simulink model "model"  (R2022b)
settings: Solver=VariableStepAuto  StartTime=0.0  StopTime=10.0  RelTol=1e-3
values from neighbouring files (symbols this model uses):
  a32 = A(3,2)    [parametry.m]
  a33 = A(3,3)    [parametry.m]
  a34 = A(3,4)    [parametry.m]
  a42 = A(4,2)    [parametry.m]
  a43 = A(4,3)    [parametry.m]
  a44 = A(4,4)    [parametry.m]
  b3 = B(3)    [parametry.m]
  b4 = B(4)    [parametry.m]
settings Model: Creator=antek  LastModifiedBy=antek

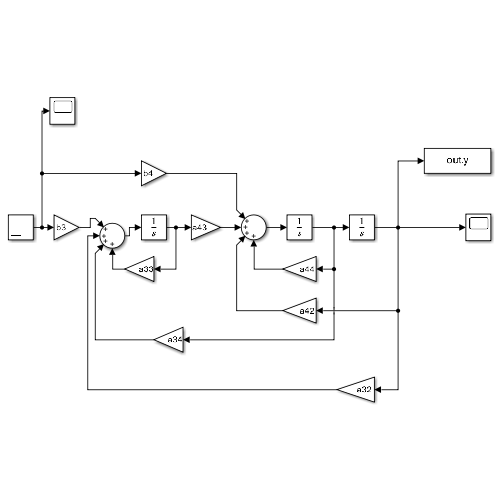
[thumbnail: Simulink's stored preview of the top-level diagram]
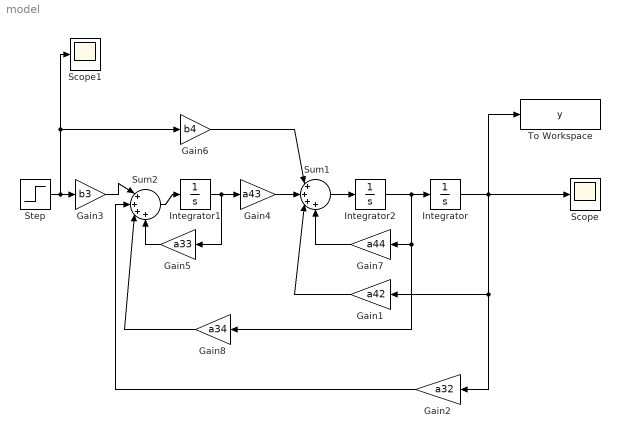
== system model ==
  Gain1 : Gain  Gain=a42
  Gain2 : Gain  Gain=a32
  Gain3 : Gain  Gain=b3
  Gain4 : Gain  Gain=a43
  Gain5 : Gain  Gain=a33
  Gain6 : Gain  Gain=b4
  Gain7 : Gain  Gain=a44
  Gain8 : Gain  Gain=a34
  Integrator : Integrator
  Integrator1 : Integrator
  Integrator2 : Integrator
  Scope : Scope
  Scope1 : Scope
  Step : Step  After=0.1  SampleTime=0
  Sum1 : Sum  Inputs=|++++
  Sum2 : Sum  Inputs=|++++
  To Workspace : ToWorkspace  VariableName=y  SaveFormat=Timeseries  SampleTime=-1
  wires:
  Gain2/1 -> Sum2/2
  Gain1/1 -> Sum1/3
  Integrator1/1 -> Gain5/1, Gain4/1
  Sum1/1 -> Integrator2/1
  Gain3/1 -> Sum2/1
  Integrator/1 -> Gain2/1, Gain1/1, Scope/1, To Workspace/1
  Sum2/1 -> Integrator1/1
  Integrator2/1 -> Gain8/1, Gain7/1, Integrator/1
  Step/1 -> Gain6/1, Scope1/1, Gain3/1
  Gain4/1 -> Sum1/2
  Gain5/1 -> Sum2/4
  Gain6/1 -> Sum1/1
  Gain7/1 -> Sum1/4
  Gain8/1 -> Sum2/3
